simulink model "practica_1"  (R2017a)
settings: Solver=VariableStepAuto  StartTime=0.0  StopTime=0.8  RelTol=1e-3
values from neighbouring files (symbols this model uses):
  C = 33e-6    (= 3.3e-05)    [Practica_1.m]
  Kd = ((1 + Kp)/(2*P*Wn)) - (R*C)    [Practica_1.m]
  Ki = ((Wn)^2)*(R*C + Kd)    [Practica_1.m]
  Kp = 0.74    [Practica_1.m]
  R = 1e3    (= 1000)    [Practica_1.m]
settings Model: Creator=lezam  LastModifiedBy=LuisCarlos

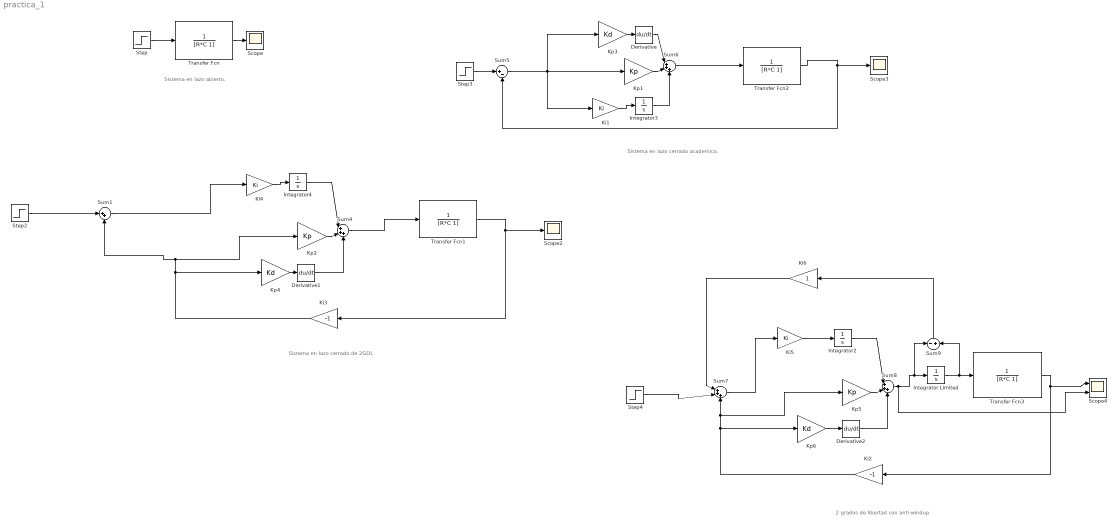
== system practica_1 ==
  note: 2 grados de libertad con anti-windup
  note: Sistema en lazo cerrado academico.
  note: Sistema en lazo cerrado de 2GDL
  note: Sistema en lazo abierto.
  Derivative : Derivative
  Derivative1 : Derivative
  Derivative2 : Derivative
  Integrator Limited : Integrator  LimitOutput=on  UpperSaturationLimit=1  LowerSaturationLimit=-1
  Integrator2 : Integrator
  Integrator3 : Integrator
  Integrator4 : Integrator
  Ki1 : Gain  Gain=Ki
  Ki2 : Gain  Gain=-1
  Ki3 : Gain  Gain=-1
  Ki4 : Gain  Gain=Ki
  Ki5 : Gain  Gain=Ki
  Ki6 : Gain
  Kp1 : Gain  Gain=Kp
  Kp2 : Gain  Gain=Kp
  Kp3 : Gain  Gain=Kd
  Kp4 : Gain  Gain=Kd
  Kp5 : Gain  Gain=Kp
  Kp6 : Gain  Gain=Kd
  Scope : Scope
  Scope2 : Scope
  Scope3 : Scope
  Scope4 : Scope  NumInputPorts=2
  Step{,2..4} (4 alike) : Step  Time=0  After=5  SampleTime=0
  Sum1 : Sum  Inputs=|++
  Sum{4,6..8} (4 alike) : Sum  Inputs=|+++
  Sum5 : Sum  Inputs=|+-
  Sum9 : Sum  Inputs=-+
  Transfer Fcn{,1..3} (4 alike) : TransferFcn  Denominator=[R*C 1]
  wires:
  Step/1 -> Transfer Fcn/1
  Transfer Fcn/1 -> Scope/1
  Sum1/1 -> Ki4/1
  Integrator4/1 -> Sum4/1
  Ki4/1 -> Integrator4/1
  Sum4/1 -> Transfer Fcn1/1
  Kp2/1 -> Sum4/2
  Kp4/1 -> Derivative1/1
  Ki3/1 -> Kp2/1, Sum1/2, Kp4/1
  Step2/1 -> Sum1/1
  Transfer Fcn1/1 -> Ki3/1, Scope2/1
  Derivative1/1 -> Sum4/3
  Integrator3/1 -> Sum6/3
  Transfer Fcn2/1 -> Sum5/2, Scope3/1
  Kp1/1 -> Sum6/2
  Derivative/1 -> Sum6/1
  Sum6/1 -> Transfer Fcn2/1
  Sum5/1 -> Kp3/1, Ki1/1, Kp1/1
  Ki1/1 -> Integrator3/1
  Kp3/1 -> Derivative/1
  Step3/1 -> Sum5/1
  Sum8/1 -> Scope4/2, Sum9/1, Integrator Limited/1
  Integrator Limited/1 -> Sum9/2, Transfer Fcn3/1
  Ki2/1 -> Sum7/3, Kp5/1, Kp6/1
  Transfer Fcn3/1 -> Ki2/1, Scope4/1
  Kp6/1 -> Derivative2/1
  Kp5/1 -> Sum8/2
  Ki5/1 -> Integrator2/1
  Integrator2/1 -> Sum8/1
  Derivative2/1 -> Sum8/3
  Sum7/1 -> Ki5/1
  Sum9/1 -> Ki6/1
  Ki6/1 -> Sum7/1
  Step4/1 -> Sum7/2
